simulink model "soc_dvbs2_fpga"  (R2025b)
settings: Solver=FixedStepDiscrete  StartTime=0.0  StopTime=0  RelTol=1e-3
InitFcn:
  | soc_dvbs2_init;
values from neighbouring files (symbols this model uses):
  Rsym = 4e6    (= 4000000)    [soc_dvbs2_init.m]
  soc_dvbs2_txPacketBits = [1 1 0 1 0 1 1 1 0 1 1 1 ... (2972 elements, 2972x1)]    [soc_dvbs2_txPacketBits.mat]
  syncWord = (dec2bin(hex2dec('AC')) - '0').'    [soc_dvbs2_init.m]
  txDataOut = txobj(frameBits(:))    [soc_dvbs2_init.m]
  txFiltCoeff = txobj.pTxFilterCoeff    [soc_dvbs2_init.m]
undefined symbols (not defined in the file or in its folder): Add, coefficientsLog, coefficientsSqrt1, coefficientsSqrt2, dataBits, designMultirateFIR, noisePow, NumBits1, NumBits2, seedsURNG1, seedsURNG2, Shift, Slope1, Slope2, soc_dvbs2_designFIRFilter, txDataOutS1, txDataOutS10, txDataOutS12, txDataOutS13, txDataOutS14, txDataOutS15, txDataOutS16, txDataOutS18, txDataOutS19, txDataOutS2, txDataOutS20, txDataOutS21, txDataOutS22, txDataOutS24, txDataOutS25, txDataOutS26, txDataOutS27, txDataOutS3, txDataOutS4, txDataOutS5, txDataOutS6, txDataOutS7, txDataOutS8, txDataOutS9
libraries: simulink x214, hdlsllib x211, dspsigops x22, dsphdlfiltering2 x8, dsphdlsigops2 x5, commseqgen3 x5, dsphdlmathfun2 x3, hwlogicconnlib x2, whdledac x2, commhdlcrc x2, whdlutilities x1, whdlmod x1
(part 11 of 12)

== system soc_dvbs2_fpga/DVBS2/DVBS2 TxRx/DVB-S2 HDL Receiver/Synchronizer and PL Header Decoder/Time Frequency and Coarse Phase Synchronizer/Fine Frequency Synchronizer/Modified L and R Algorithm/L and R Algorithm 18 point/Compute R(m) for 1 to 6/Compute R(m)_1/Complex Multiplier ==
  In1 : Inport
  In2 : Inport  Port=2
  AddADn : Sum  Inputs=++|  OutDataTypeStr=Inherit: Same as first input
  AddAUp : Sum  Inputs=|+-  OutDataTypeStr=Inherit: Same as first input
  AddBCtr : Sum  Inputs=+|+
  AddBDn : Sum  Inputs=|+-
  AddBUp : Sum  Inputs=++|
  Complex to Real-Imag : ComplexToRealImag
  Complex to Real-Imag1 : ComplexToRealImag
  Delay{1..5,8..20} (18 alike) : Delay  DelayLength=1
  Delay{6..7,21..27} (9 alike) : Delay
  Product : Product
  Product1 : Product
  Product2 : Product
  Real-Imag to Complex : RealImagToComplex
  Out1 : Outport  VectorParamsAs1DForOutWhenUnconnected=off
  wires:
  Delay27/1 -> Delay18/1
  Delay26/1 -> Delay17/1
  Delay25/1 -> Delay16/1
  Delay24/1 -> Product2/2
  Delay23/1 -> Product2/1
  Delay22/1 -> Product1/2
  Delay21/1 -> Product1/1
  Delay7/1 -> Product/2
  Delay6/1 -> Product/1
  In1/1 -> Complex to Real-Imag/1
  In2/1 -> Complex to Real-Imag1/1
  Complex to Real-Imag1/1 -> [RE2]
  Complex to Real-Imag1/2 -> [IM2]
  [IM2] -> Delay10/1
  [RE2] -> Delay9/1
  Complex to Real-Imag/1 -> Delay11/1
  AddBUp/1 -> Delay8/1
  [RE2] -> Delay14/1
  [IM2] -> Delay15/1
  AddBDn/1 -> Delay5/1
  Complex to Real-Imag/2 -> Delay13/1
  AddBCtr/1 -> Delay2/1
  [IM2] -> Delay12/1
  AddADn/1 -> Delay20/1
  AddAUp/1 -> Delay19/1
  Real-Imag to Complex/1 -> Out1/1
  Product/1 -> Delay25/1
  Product1/1 -> Delay26/1
  Product2/1 -> Delay27/1
  Delay5/1 -> Delay24/1
  Delay4/1 -> Delay23/1
  Delay3/1 -> Delay22/1
  Delay2/1 -> Delay21/1
  Delay8/1 -> Delay6/1
  Delay9/1 -> AddBUp/1
  Delay10/1 -> AddBUp/2
  Delay14/1 -> AddBDn/1
  Delay15/1 -> AddBDn/2
  Delay16/1 -> AddAUp/1
  Delay17/1 -> AddADn/1, AddAUp/2
  Delay18/1 -> AddADn/2
  Delay19/1 -> Real-Imag to Complex/1
  Delay20/1 -> Real-Imag to Complex/2
  Delay1/1 -> Delay7/1
  Delay11/1 -> AddBCtr/1, Delay1/1
  Delay12/1 -> Delay3/1
  Delay13/1 -> AddBCtr/2, Delay4/1

== system soc_dvbs2_fpga/DVBS2/DVBS2 TxRx/DVB-S2 HDL Receiver/Synchronizer and PL Header Decoder/Time Frequency and Coarse Phase Synchronizer/Fine Frequency Synchronizer/Modified L and R Algorithm/L and R Algorithm 18 point/Compute R(m) for 1 to 6/Compute R(m)_2/Complex Multiplier ==
  In1 : Inport
  In2 : Inport  Port=2
  AddADn : Sum  Inputs=++|  OutDataTypeStr=Inherit: Same as first input
  AddAUp : Sum  Inputs=|+-  OutDataTypeStr=Inherit: Same as first input
  AddBCtr : Sum  Inputs=+|+
  AddBDn : Sum  Inputs=|+-
  AddBUp : Sum  Inputs=++|
  Complex to Real-Imag : ComplexToRealImag
  Complex to Real-Imag1 : ComplexToRealImag
  Delay{1..5,8..20} (18 alike) : Delay  DelayLength=1
  Delay{6..7,21..27} (9 alike) : Delay
  Product : Product
  Product1 : Product
  Product2 : Product
  Real-Imag to Complex : RealImagToComplex
  Out1 : Outport  VectorParamsAs1DForOutWhenUnconnected=off
  wires:
  Delay13/1 -> Delay4/1, AddBCtr/2
  Delay12/1 -> Delay3/1
  Delay11/1 -> Delay1/1, AddBCtr/1
  Delay1/1 -> Delay7/1
  Delay20/1 -> Real-Imag to Complex/2
  Delay19/1 -> Real-Imag to Complex/1
  Delay18/1 -> AddADn/2
  Delay17/1 -> AddAUp/2, AddADn/1
  Delay16/1 -> AddAUp/1
  Delay15/1 -> AddBDn/2
  Delay14/1 -> AddBDn/1
  Delay10/1 -> AddBUp/2
  Delay9/1 -> AddBUp/1
  Delay8/1 -> Delay6/1
  Delay2/1 -> Delay21/1
  Delay3/1 -> Delay22/1
  Delay4/1 -> Delay23/1
  Delay5/1 -> Delay24/1
  Product2/1 -> Delay27/1
  Product1/1 -> Delay26/1
  Product/1 -> Delay25/1
  Real-Imag to Complex/1 -> Out1/1
  AddAUp/1 -> Delay19/1
  AddADn/1 -> Delay20/1
  [IM2] -> Delay12/1
  AddBCtr/1 -> Delay2/1
  Complex to Real-Imag/2 -> Delay13/1
  AddBDn/1 -> Delay5/1
  [IM2] -> Delay15/1
  [RE2] -> Delay14/1
  AddBUp/1 -> Delay8/1
  Complex to Real-Imag/1 -> Delay11/1
  [RE2] -> Delay9/1
  [IM2] -> Delay10/1
  Complex to Real-Imag1/2 -> [IM2]
  Complex to Real-Imag1/1 -> [RE2]
  In2/1 -> Complex to Real-Imag1/1
  In1/1 -> Complex to Real-Imag/1
  Delay6/1 -> Product/1
  Delay7/1 -> Product/2
  Delay21/1 -> Product1/1
  Delay22/1 -> Product1/2
  Delay23/1 -> Product2/1
  Delay24/1 -> Product2/2
  Delay25/1 -> Delay16/1
  Delay26/1 -> Delay17/1
  Delay27/1 -> Delay18/1

== system soc_dvbs2_fpga/DVBS2/DVBS2 TxRx/DVB-S2 HDL Receiver/Synchronizer and PL Header Decoder/Time Frequency and Coarse Phase Synchronizer/Fine Frequency Synchronizer/Modified L and R Algorithm/L and R Algorithm 18 point/Compute R(m) for 1 to 6/Compute R(m)_3/Complex Multiplier ==
  In1 : Inport
  In2 : Inport  Port=2
  AddADn : Sum  Inputs=++|  OutDataTypeStr=Inherit: Same as first input
  AddAUp : Sum  Inputs=|+-  OutDataTypeStr=Inherit: Same as first input
  AddBCtr : Sum  Inputs=+|+
  AddBDn : Sum  Inputs=|+-
  AddBUp : Sum  Inputs=++|
  Complex to Real-Imag : ComplexToRealImag
  Complex to Real-Imag1 : ComplexToRealImag
  Delay{1..5,8..20} (18 alike) : Delay  DelayLength=1
  Delay{6..7,21..27} (9 alike) : Delay
  Product : Product
  Product1 : Product
  Product2 : Product
  Real-Imag to Complex : RealImagToComplex
  Out1 : Outport  VectorParamsAs1DForOutWhenUnconnected=off
  wires:
  Delay27/1 -> Delay18/1
  Delay26/1 -> Delay17/1
  Delay25/1 -> Delay16/1
  Delay24/1 -> Product2/2
  Delay23/1 -> Product2/1
  Delay22/1 -> Product1/2
  Delay21/1 -> Product1/1
  Delay7/1 -> Product/2
  Delay6/1 -> Product/1
  In1/1 -> Complex to Real-Imag/1
  In2/1 -> Complex to Real-Imag1/1
  Complex to Real-Imag1/1 -> [RE2]
  Complex to Real-Imag1/2 -> [IM2]
  [IM2] -> Delay10/1
  [RE2] -> Delay9/1
  Complex to Real-Imag/1 -> Delay11/1
  AddBUp/1 -> Delay8/1
  [RE2] -> Delay14/1
  [IM2] -> Delay15/1
  AddBDn/1 -> Delay5/1
  Complex to Real-Imag/2 -> Delay13/1
  AddBCtr/1 -> Delay2/1
  [IM2] -> Delay12/1
  AddADn/1 -> Delay20/1
  AddAUp/1 -> Delay19/1
  Real-Imag to Complex/1 -> Out1/1
  Product/1 -> Delay25/1
  Product1/1 -> Delay26/1
  Product2/1 -> Delay27/1
  Delay5/1 -> Delay24/1
  Delay4/1 -> Delay23/1
  Delay3/1 -> Delay22/1
  Delay2/1 -> Delay21/1
  Delay8/1 -> Delay6/1
  Delay9/1 -> AddBUp/1
  Delay10/1 -> AddBUp/2
  Delay14/1 -> AddBDn/1
  Delay15/1 -> AddBDn/2
  Delay16/1 -> AddAUp/1
  Delay17/1 -> AddADn/1, AddAUp/2
  Delay18/1 -> AddADn/2
  Delay19/1 -> Real-Imag to Complex/1
  Delay20/1 -> Real-Imag to Complex/2
  Delay1/1 -> Delay7/1
  Delay11/1 -> AddBCtr/1, Delay1/1
  Delay12/1 -> Delay3/1
  Delay13/1 -> AddBCtr/2, Delay4/1

== system soc_dvbs2_fpga/DVBS2/DVBS2 TxRx/DVB-S2 HDL Receiver/Synchronizer and PL Header Decoder/Time Frequency and Coarse Phase Synchronizer/Fine Frequency Synchronizer/Modified L and R Algorithm/L and R Algorithm 18 point/Compute R(m) for 1 to 6/Compute R(m)_4/Complex Multiplier ==
  In1 : Inport
  In2 : Inport  Port=2
  AddADn : Sum  Inputs=++|  OutDataTypeStr=Inherit: Same as first input
  AddAUp : Sum  Inputs=|+-  OutDataTypeStr=Inherit: Same as first input
  AddBCtr : Sum  Inputs=+|+
  AddBDn : Sum  Inputs=|+-
  AddBUp : Sum  Inputs=++|
  Complex to Real-Imag : ComplexToRealImag
  Complex to Real-Imag1 : ComplexToRealImag
  Delay{1..5,8..20} (18 alike) : Delay  DelayLength=1
  Delay{6..7,21..27} (9 alike) : Delay
  Product : Product
  Product1 : Product
  Product2 : Product
  Real-Imag to Complex : RealImagToComplex
  Out1 : Outport  VectorParamsAs1DForOutWhenUnconnected=off
  wires:
  Delay13/1 -> Delay4/1, AddBCtr/2
  Delay12/1 -> Delay3/1
  Delay11/1 -> Delay1/1, AddBCtr/1
  Delay1/1 -> Delay7/1
  Delay20/1 -> Real-Imag to Complex/2
  Delay19/1 -> Real-Imag to Complex/1
  Delay18/1 -> AddADn/2
  Delay17/1 -> AddAUp/2, AddADn/1
  Delay16/1 -> AddAUp/1
  Delay15/1 -> AddBDn/2
  Delay14/1 -> AddBDn/1
  Delay10/1 -> AddBUp/2
  Delay9/1 -> AddBUp/1
  Delay8/1 -> Delay6/1
  Delay2/1 -> Delay21/1
  Delay3/1 -> Delay22/1
  Delay4/1 -> Delay23/1
  Delay5/1 -> Delay24/1
  Product2/1 -> Delay27/1
  Product1/1 -> Delay26/1
  Product/1 -> Delay25/1
  Real-Imag to Complex/1 -> Out1/1
  AddAUp/1 -> Delay19/1
  AddADn/1 -> Delay20/1
  [IM2] -> Delay12/1
  AddBCtr/1 -> Delay2/1
  Complex to Real-Imag/2 -> Delay13/1
  AddBDn/1 -> Delay5/1
  [IM2] -> Delay15/1
  [RE2] -> Delay14/1
  AddBUp/1 -> Delay8/1
  Complex to Real-Imag/1 -> Delay11/1
  [RE2] -> Delay9/1
  [IM2] -> Delay10/1
  Complex to Real-Imag1/2 -> [IM2]
  Complex to Real-Imag1/1 -> [RE2]
  In2/1 -> Complex to Real-Imag1/1
  In1/1 -> Complex to Real-Imag/1
  Delay6/1 -> Product/1
  Delay7/1 -> Product/2
  Delay21/1 -> Product1/1
  Delay22/1 -> Product1/2
  Delay23/1 -> Product2/1
  Delay24/1 -> Product2/2
  Delay25/1 -> Delay16/1
  Delay26/1 -> Delay17/1
  Delay27/1 -> Delay18/1

== system soc_dvbs2_fpga/DVBS2/DVBS2 TxRx/DVB-S2 HDL Receiver/Synchronizer and PL Header Decoder/Time Frequency and Coarse Phase Synchronizer/Fine Frequency Synchronizer/Modified L and R Algorithm/L and R Algorithm 18 point/Compute R(m) for 1 to 6/Compute R(m)_5/Complex Multiplier ==
  In1 : Inport
  In2 : Inport  Port=2
  AddADn : Sum  Inputs=++|  OutDataTypeStr=Inherit: Same as first input
  AddAUp : Sum  Inputs=|+-  OutDataTypeStr=Inherit: Same as first input
  AddBCtr : Sum  Inputs=+|+
  AddBDn : Sum  Inputs=|+-
  AddBUp : Sum  Inputs=++|
  Complex to Real-Imag : ComplexToRealImag
  Complex to Real-Imag1 : ComplexToRealImag
  Delay{1..5,8..20} (18 alike) : Delay  DelayLength=1
  Delay{6..7,21..27} (9 alike) : Delay
  Product : Product
  Product1 : Product
  Product2 : Product
  Real-Imag to Complex : RealImagToComplex
  Out1 : Outport  VectorParamsAs1DForOutWhenUnconnected=off
  wires:
  Delay27/1 -> Delay18/1
  Delay26/1 -> Delay17/1
  Delay25/1 -> Delay16/1
  Delay24/1 -> Product2/2
  Delay23/1 -> Product2/1
  Delay22/1 -> Product1/2
  Delay21/1 -> Product1/1
  Delay7/1 -> Product/2
  Delay6/1 -> Product/1
  In1/1 -> Complex to Real-Imag/1
  In2/1 -> Complex to Real-Imag1/1
  Complex to Real-Imag1/1 -> [RE2]
  Complex to Real-Imag1/2 -> [IM2]
  [IM2] -> Delay10/1
  [RE2] -> Delay9/1
  Complex to Real-Imag/1 -> Delay11/1
  AddBUp/1 -> Delay8/1
  [RE2] -> Delay14/1
  [IM2] -> Delay15/1
  AddBDn/1 -> Delay5/1
  Complex to Real-Imag/2 -> Delay13/1
  AddBCtr/1 -> Delay2/1
  [IM2] -> Delay12/1
  AddADn/1 -> Delay20/1
  AddAUp/1 -> Delay19/1
  Real-Imag to Complex/1 -> Out1/1
  Product/1 -> Delay25/1
  Product1/1 -> Delay26/1
  Product2/1 -> Delay27/1
  Delay5/1 -> Delay24/1
  Delay4/1 -> Delay23/1
  Delay3/1 -> Delay22/1
  Delay2/1 -> Delay21/1
  Delay8/1 -> Delay6/1
  Delay9/1 -> AddBUp/1
  Delay10/1 -> AddBUp/2
  Delay14/1 -> AddBDn/1
  Delay15/1 -> AddBDn/2
  Delay16/1 -> AddAUp/1
  Delay17/1 -> AddADn/1, AddAUp/2
  Delay18/1 -> AddADn/2
  Delay19/1 -> Real-Imag to Complex/1
  Delay20/1 -> Real-Imag to Complex/2
  Delay1/1 -> Delay7/1
  Delay11/1 -> AddBCtr/1, Delay1/1
  Delay12/1 -> Delay3/1
  Delay13/1 -> AddBCtr/2, Delay4/1

== system soc_dvbs2_fpga/DVBS2/DVBS2 TxRx/DVB-S2 HDL Receiver/Synchronizer and PL Header Decoder/Time Frequency and Coarse Phase Synchronizer/Fine Frequency Synchronizer/Modified L and R Algorithm/L and R Algorithm 18 point/Compute R(m) for 1 to 6/Compute R(m)_6/Complex Multiplier ==
  In1 : Inport
  In2 : Inport  Port=2
  AddADn : Sum  Inputs=++|  OutDataTypeStr=Inherit: Same as first input
  AddAUp : Sum  Inputs=|+-  OutDataTypeStr=Inherit: Same as first input
  AddBCtr : Sum  Inputs=+|+
  AddBDn : Sum  Inputs=|+-
  AddBUp : Sum  Inputs=++|
  Complex to Real-Imag : ComplexToRealImag
  Complex to Real-Imag1 : ComplexToRealImag
  Delay{1..5,8..20} (18 alike) : Delay  DelayLength=1
  Delay{6..7,21..27} (9 alike) : Delay
  Product : Product
  Product1 : Product
  Product2 : Product
  Real-Imag to Complex : RealImagToComplex
  Out1 : Outport  VectorParamsAs1DForOutWhenUnconnected=off
  wires:
  Delay13/1 -> Delay4/1, AddBCtr/2
  Delay12/1 -> Delay3/1
  Delay11/1 -> Delay1/1, AddBCtr/1
  Delay1/1 -> Delay7/1
  Delay20/1 -> Real-Imag to Complex/2
  Delay19/1 -> Real-Imag to Complex/1
  Delay18/1 -> AddADn/2
  Delay17/1 -> AddAUp/2, AddADn/1
  Delay16/1 -> AddAUp/1
  Delay15/1 -> AddBDn/2
  Delay14/1 -> AddBDn/1
  Delay10/1 -> AddBUp/2
  Delay9/1 -> AddBUp/1
  Delay8/1 -> Delay6/1
  Delay2/1 -> Delay21/1
  Delay3/1 -> Delay22/1
  Delay4/1 -> Delay23/1
  Delay5/1 -> Delay24/1
  Product2/1 -> Delay27/1
  Product1/1 -> Delay26/1
  Product/1 -> Delay25/1
  Real-Imag to Complex/1 -> Out1/1
  AddAUp/1 -> Delay19/1
  AddADn/1 -> Delay20/1
  [IM2] -> Delay12/1
  AddBCtr/1 -> Delay2/1
  Complex to Real-Imag/2 -> Delay13/1
  AddBDn/1 -> Delay5/1
  [IM2] -> Delay15/1
  [RE2] -> Delay14/1
  AddBUp/1 -> Delay8/1
  Complex to Real-Imag/1 -> Delay11/1
  [RE2] -> Delay9/1
  [IM2] -> Delay10/1
  Complex to Real-Imag1/2 -> [IM2]
  Complex to Real-Imag1/1 -> [RE2]
  In2/1 -> Complex to Real-Imag1/1
  In1/1 -> Complex to Real-Imag/1
  Delay6/1 -> Product/1
  Delay7/1 -> Product/2
  Delay21/1 -> Product1/1
  Delay22/1 -> Product1/2
  Delay23/1 -> Product2/1
  Delay24/1 -> Product2/2
  Delay25/1 -> Delay16/1
  Delay26/1 -> Delay17/1
  Delay27/1 -> Delay18/1

== system soc_dvbs2_fpga/DVBS2/DVBS2 TxRx/DVB-S2 HDL Receiver/Synchronizer and PL Header Decoder/Time Frequency and Coarse Phase Synchronizer/Fine Frequency Synchronizer/Modified L and R Algorithm/L and R Algorithm 18 point/Compute R(m) for 13 to 18/Compute R(m)_1/Complex Multiplier ==
  In1 : Inport
  In2 : Inport  Port=2
  AddADn : Sum  Inputs=++|  OutDataTypeStr=Inherit: Same as first input
  AddAUp : Sum  Inputs=|+-  OutDataTypeStr=Inherit: Same as first input
  AddBCtr : Sum  Inputs=+|+
  AddBDn : Sum  Inputs=|+-
  AddBUp : Sum  Inputs=++|
  Complex to Real-Imag : ComplexToRealImag
  Complex to Real-Imag1 : ComplexToRealImag
  Delay{1..5,8..20} (18 alike) : Delay  DelayLength=1
  Delay{6..7,21..27} (9 alike) : Delay
  Product : Product
  Product1 : Product
  Product2 : Product
  Real-Imag to Complex : RealImagToComplex
  Out1 : Outport  VectorParamsAs1DForOutWhenUnconnected=off
  wires:
  Delay27/1 -> Delay18/1
  Delay26/1 -> Delay17/1
  Delay25/1 -> Delay16/1
  Delay24/1 -> Product2/2
  Delay23/1 -> Product2/1
  Delay22/1 -> Product1/2
  Delay21/1 -> Product1/1
  Delay7/1 -> Product/2
  Delay6/1 -> Product/1
  In1/1 -> Complex to Real-Imag/1
  In2/1 -> Complex to Real-Imag1/1
  Complex to Real-Imag1/1 -> [RE2]
  Complex to Real-Imag1/2 -> [IM2]
  [IM2] -> Delay10/1
  [RE2] -> Delay9/1
  Complex to Real-Imag/1 -> Delay11/1
  AddBUp/1 -> Delay8/1
  [RE2] -> Delay14/1
  [IM2] -> Delay15/1
  AddBDn/1 -> Delay5/1
  Complex to Real-Imag/2 -> Delay13/1
  AddBCtr/1 -> Delay2/1
  [IM2] -> Delay12/1
  AddADn/1 -> Delay20/1
  AddAUp/1 -> Delay19/1
  Real-Imag to Complex/1 -> Out1/1
  Product/1 -> Delay25/1
  Product1/1 -> Delay26/1
  Product2/1 -> Delay27/1
  Delay5/1 -> Delay24/1
  Delay4/1 -> Delay23/1
  Delay3/1 -> Delay22/1
  Delay2/1 -> Delay21/1
  Delay8/1 -> Delay6/1
  Delay9/1 -> AddBUp/1
  Delay10/1 -> AddBUp/2
  Delay14/1 -> AddBDn/1
  Delay15/1 -> AddBDn/2
  Delay16/1 -> AddAUp/1
  Delay17/1 -> AddADn/1, AddAUp/2
  Delay18/1 -> AddADn/2
  Delay19/1 -> Real-Imag to Complex/1
  Delay20/1 -> Real-Imag to Complex/2
  Delay1/1 -> Delay7/1
  Delay11/1 -> AddBCtr/1, Delay1/1
  Delay12/1 -> Delay3/1
  Delay13/1 -> AddBCtr/2, Delay4/1

== system soc_dvbs2_fpga/DVBS2/DVBS2 TxRx/DVB-S2 HDL Receiver/Synchronizer and PL Header Decoder/Time Frequency and Coarse Phase Synchronizer/Fine Frequency Synchronizer/Modified L and R Algorithm/L and R Algorithm 18 point/Compute R(m) for 13 to 18/Compute R(m)_2/Complex Multiplier ==
  In1 : Inport
  In2 : Inport  Port=2
  AddADn : Sum  Inputs=++|  OutDataTypeStr=Inherit: Same as first input
  AddAUp : Sum  Inputs=|+-  OutDataTypeStr=Inherit: Same as first input
  AddBCtr : Sum  Inputs=+|+
  AddBDn : Sum  Inputs=|+-
  AddBUp : Sum  Inputs=++|
  Complex to Real-Imag : ComplexToRealImag
  Complex to Real-Imag1 : ComplexToRealImag
  Delay{1..5,8..20} (18 alike) : Delay  DelayLength=1
  Delay{6..7,21..27} (9 alike) : Delay
  Product : Product
  Product1 : Product
  Product2 : Product
  Real-Imag to Complex : RealImagToComplex
  Out1 : Outport  VectorParamsAs1DForOutWhenUnconnected=off
  wires:
  Delay13/1 -> Delay4/1, AddBCtr/2
  Delay12/1 -> Delay3/1
  Delay11/1 -> Delay1/1, AddBCtr/1
  Delay1/1 -> Delay7/1
  Delay20/1 -> Real-Imag to Complex/2
  Delay19/1 -> Real-Imag to Complex/1
  Delay18/1 -> AddADn/2
  Delay17/1 -> AddAUp/2, AddADn/1
  Delay16/1 -> AddAUp/1
  Delay15/1 -> AddBDn/2
  Delay14/1 -> AddBDn/1
  Delay10/1 -> AddBUp/2
  Delay9/1 -> AddBUp/1
  Delay8/1 -> Delay6/1
  Delay2/1 -> Delay21/1
  Delay3/1 -> Delay22/1
  Delay4/1 -> Delay23/1
  Delay5/1 -> Delay24/1
  Product2/1 -> Delay27/1
  Product1/1 -> Delay26/1
  Product/1 -> Delay25/1
  Real-Imag to Complex/1 -> Out1/1
  AddAUp/1 -> Delay19/1
  AddADn/1 -> Delay20/1
  [IM2] -> Delay12/1
  AddBCtr/1 -> Delay2/1
  Complex to Real-Imag/2 -> Delay13/1
  AddBDn/1 -> Delay5/1
  [IM2] -> Delay15/1
  [RE2] -> Delay14/1
  AddBUp/1 -> Delay8/1
  Complex to Real-Imag/1 -> Delay11/1
  [RE2] -> Delay9/1
  [IM2] -> Delay10/1
  Complex to Real-Imag1/2 -> [IM2]
  Complex to Real-Imag1/1 -> [RE2]
  In2/1 -> Complex to Real-Imag1/1
  In1/1 -> Complex to Real-Imag/1
  Delay6/1 -> Product/1
  Delay7/1 -> Product/2
  Delay21/1 -> Product1/1
  Delay22/1 -> Product1/2
  Delay23/1 -> Product2/1
  Delay24/1 -> Product2/2
  Delay25/1 -> Delay16/1
  Delay26/1 -> Delay17/1
  Delay27/1 -> Delay18/1

== system soc_dvbs2_fpga/DVBS2/DVBS2 TxRx/DVB-S2 HDL Receiver/Synchronizer and PL Header Decoder/Time Frequency and Coarse Phase Synchronizer/Fine Frequency Synchronizer/Modified L and R Algorithm/L and R Algorithm 18 point/Compute R(m) for 13 to 18/Compute R(m)_3/Complex Multiplier ==
  In1 : Inport
  In2 : Inport  Port=2
  AddADn : Sum  Inputs=++|  OutDataTypeStr=Inherit: Same as first input
  AddAUp : Sum  Inputs=|+-  OutDataTypeStr=Inherit: Same as first input
  AddBCtr : Sum  Inputs=+|+
  AddBDn : Sum  Inputs=|+-
  AddBUp : Sum  Inputs=++|
  Complex to Real-Imag : ComplexToRealImag
  Complex to Real-Imag1 : ComplexToRealImag
  Delay{1..5,8..20} (18 alike) : Delay  DelayLength=1
  Delay{6..7,21..27} (9 alike) : Delay
  Product : Product
  Product1 : Product
  Product2 : Product
  Real-Imag to Complex : RealImagToComplex
  Out1 : Outport  VectorParamsAs1DForOutWhenUnconnected=off
  wires:
  Delay27/1 -> Delay18/1
  Delay26/1 -> Delay17/1
  Delay25/1 -> Delay16/1
  Delay24/1 -> Product2/2
  Delay23/1 -> Product2/1
  Delay22/1 -> Product1/2
  Delay21/1 -> Product1/1
  Delay7/1 -> Product/2
  Delay6/1 -> Product/1
  In1/1 -> Complex to Real-Imag/1
  In2/1 -> Complex to Real-Imag1/1
  Complex to Real-Imag1/1 -> [RE2]
  Complex to Real-Imag1/2 -> [IM2]
  [IM2] -> Delay10/1
  [RE2] -> Delay9/1
  Complex to Real-Imag/1 -> Delay11/1
  AddBUp/1 -> Delay8/1
  [RE2] -> Delay14/1
  [IM2] -> Delay15/1
  AddBDn/1 -> Delay5/1
  Complex to Real-Imag/2 -> Delay13/1
  AddBCtr/1 -> Delay2/1
  [IM2] -> Delay12/1
  AddADn/1 -> Delay20/1
  AddAUp/1 -> Delay19/1
  Real-Imag to Complex/1 -> Out1/1
  Product/1 -> Delay25/1
  Product1/1 -> Delay26/1
  Product2/1 -> Delay27/1
  Delay5/1 -> Delay24/1
  Delay4/1 -> Delay23/1
  Delay3/1 -> Delay22/1
  Delay2/1 -> Delay21/1
  Delay8/1 -> Delay6/1
  Delay9/1 -> AddBUp/1
  Delay10/1 -> AddBUp/2
  Delay14/1 -> AddBDn/1
  Delay15/1 -> AddBDn/2
  Delay16/1 -> AddAUp/1
  Delay17/1 -> AddADn/1, AddAUp/2
  Delay18/1 -> AddADn/2
  Delay19/1 -> Real-Imag to Complex/1
  Delay20/1 -> Real-Imag to Complex/2
  Delay1/1 -> Delay7/1
  Delay11/1 -> AddBCtr/1, Delay1/1
  Delay12/1 -> Delay3/1
  Delay13/1 -> AddBCtr/2, Delay4/1

== system soc_dvbs2_fpga/DVBS2/DVBS2 TxRx/DVB-S2 HDL Receiver/Synchronizer and PL Header Decoder/Time Frequency and Coarse Phase Synchronizer/Fine Frequency Synchronizer/Modified L and R Algorithm/L and R Algorithm 18 point/Compute R(m) for 13 to 18/Compute R(m)_4/Complex Multiplier ==
  In1 : Inport
  In2 : Inport  Port=2
  AddADn : Sum  Inputs=++|  OutDataTypeStr=Inherit: Same as first input
  AddAUp : Sum  Inputs=|+-  OutDataTypeStr=Inherit: Same as first input
  AddBCtr : Sum  Inputs=+|+
  AddBDn : Sum  Inputs=|+-
  AddBUp : Sum  Inputs=++|
  Complex to Real-Imag : ComplexToRealImag
  Complex to Real-Imag1 : ComplexToRealImag
  Delay{1..5,8..20} (18 alike) : Delay  DelayLength=1
  Delay{6..7,21..27} (9 alike) : Delay
  Product : Product
  Product1 : Product
  Product2 : Product
  Real-Imag to Complex : RealImagToComplex
  Out1 : Outport  VectorParamsAs1DForOutWhenUnconnected=off
  wires:
  Delay13/1 -> Delay4/1, AddBCtr/2
  Delay12/1 -> Delay3/1
  Delay11/1 -> Delay1/1, AddBCtr/1
  Delay1/1 -> Delay7/1
  Delay20/1 -> Real-Imag to Complex/2
  Delay19/1 -> Real-Imag to Complex/1
  Delay18/1 -> AddADn/2
  Delay17/1 -> AddAUp/2, AddADn/1
  Delay16/1 -> AddAUp/1
  Delay15/1 -> AddBDn/2
  Delay14/1 -> AddBDn/1
  Delay10/1 -> AddBUp/2
  Delay9/1 -> AddBUp/1
  Delay8/1 -> Delay6/1
  Delay2/1 -> Delay21/1
  Delay3/1 -> Delay22/1
  Delay4/1 -> Delay23/1
  Delay5/1 -> Delay24/1
  Product2/1 -> Delay27/1
  Product1/1 -> Delay26/1
  Product/1 -> Delay25/1
  Real-Imag to Complex/1 -> Out1/1
  AddAUp/1 -> Delay19/1
  AddADn/1 -> Delay20/1
  [IM2] -> Delay12/1
  AddBCtr/1 -> Delay2/1
  Complex to Real-Imag/2 -> Delay13/1
  AddBDn/1 -> Delay5/1
  [IM2] -> Delay15/1
  [RE2] -> Delay14/1
  AddBUp/1 -> Delay8/1
  Complex to Real-Imag/1 -> Delay11/1
  [RE2] -> Delay9/1
  [IM2] -> Delay10/1
  Complex to Real-Imag1/2 -> [IM2]
  Complex to Real-Imag1/1 -> [RE2]
  In2/1 -> Complex to Real-Imag1/1
  In1/1 -> Complex to Real-Imag/1
  Delay6/1 -> Product/1
  Delay7/1 -> Product/2
  Delay21/1 -> Product1/1
  Delay22/1 -> Product1/2
  Delay23/1 -> Product2/1
  Delay24/1 -> Product2/2
  Delay25/1 -> Delay16/1
  Delay26/1 -> Delay17/1
  Delay27/1 -> Delay18/1

== system soc_dvbs2_fpga/DVBS2/DVBS2 TxRx/DVB-S2 HDL Receiver/Synchronizer and PL Header Decoder/Time Frequency and Coarse Phase Synchronizer/Fine Frequency Synchronizer/Modified L and R Algorithm/L and R Algorithm 18 point/Compute R(m) for 13 to 18/Compute R(m)_5/Complex Multiplier ==
  In1 : Inport
  In2 : Inport  Port=2
  AddADn : Sum  Inputs=++|  OutDataTypeStr=Inherit: Same as first input
  AddAUp : Sum  Inputs=|+-  OutDataTypeStr=Inherit: Same as first input
  AddBCtr : Sum  Inputs=+|+
  AddBDn : Sum  Inputs=|+-
  AddBUp : Sum  Inputs=++|
  Complex to Real-Imag : ComplexToRealImag
  Complex to Real-Imag1 : ComplexToRealImag
  Delay{1..5,8..20} (18 alike) : Delay  DelayLength=1
  Delay{6..7,21..27} (9 alike) : Delay
  Product : Product
  Product1 : Product
  Product2 : Product
  Real-Imag to Complex : RealImagToComplex
  Out1 : Outport  VectorParamsAs1DForOutWhenUnconnected=off
  wires:
  Delay27/1 -> Delay18/1
  Delay26/1 -> Delay17/1
  Delay25/1 -> Delay16/1
  Delay24/1 -> Product2/2
  Delay23/1 -> Product2/1
  Delay22/1 -> Product1/2
  Delay21/1 -> Product1/1
  Delay7/1 -> Product/2
  Delay6/1 -> Product/1
  In1/1 -> Complex to Real-Imag/1
  In2/1 -> Complex to Real-Imag1/1
  Complex to Real-Imag1/1 -> [RE2]
  Complex to Real-Imag1/2 -> [IM2]
  [IM2] -> Delay10/1
  [RE2] -> Delay9/1
  Complex to Real-Imag/1 -> Delay11/1
  AddBUp/1 -> Delay8/1
  [RE2] -> Delay14/1
  [IM2] -> Delay15/1
  AddBDn/1 -> Delay5/1
  Complex to Real-Imag/2 -> Delay13/1
  AddBCtr/1 -> Delay2/1
  [IM2] -> Delay12/1
  AddADn/1 -> Delay20/1
  AddAUp/1 -> Delay19/1
  Real-Imag to Complex/1 -> Out1/1
  Product/1 -> Delay25/1
  Product1/1 -> Delay26/1
  Product2/1 -> Delay27/1
  Delay5/1 -> Delay24/1
  Delay4/1 -> Delay23/1
  Delay3/1 -> Delay22/1
  Delay2/1 -> Delay21/1
  Delay8/1 -> Delay6/1
  Delay9/1 -> AddBUp/1
  Delay10/1 -> AddBUp/2
  Delay14/1 -> AddBDn/1
  Delay15/1 -> AddBDn/2
  Delay16/1 -> AddAUp/1
  Delay17/1 -> AddADn/1, AddAUp/2
  Delay18/1 -> AddADn/2
  Delay19/1 -> Real-Imag to Complex/1
  Delay20/1 -> Real-Imag to Complex/2
  Delay1/1 -> Delay7/1
  Delay11/1 -> AddBCtr/1, Delay1/1
  Delay12/1 -> Delay3/1
  Delay13/1 -> AddBCtr/2, Delay4/1

== system soc_dvbs2_fpga/DVBS2/DVBS2 TxRx/DVB-S2 HDL Receiver/Synchronizer and PL Header Decoder/Time Frequency and Coarse Phase Synchronizer/Fine Frequency Synchronizer/Modified L and R Algorithm/L and R Algorithm 18 point/Compute R(m) for 13 to 18/Compute R(m)_6/Complex Multiplier ==
  In1 : Inport
  In2 : Inport  Port=2
  AddADn : Sum  Inputs=++|  OutDataTypeStr=Inherit: Same as first input
  AddAUp : Sum  Inputs=|+-  OutDataTypeStr=Inherit: Same as first input
  AddBCtr : Sum  Inputs=+|+
  AddBDn : Sum  Inputs=|+-
  AddBUp : Sum  Inputs=++|
  Complex to Real-Imag : ComplexToRealImag
  Complex to Real-Imag1 : ComplexToRealImag
  Delay{1..5,8..20} (18 alike) : Delay  DelayLength=1
  Delay{6..7,21..27} (9 alike) : Delay
  Product : Product
  Product1 : Product
  Product2 : Product
  Real-Imag to Complex : RealImagToComplex
  Out1 : Outport  VectorParamsAs1DForOutWhenUnconnected=off
  wires:
  Delay13/1 -> Delay4/1, AddBCtr/2
  Delay12/1 -> Delay3/1
  Delay11/1 -> Delay1/1, AddBCtr/1
  Delay1/1 -> Delay7/1
  Delay20/1 -> Real-Imag to Complex/2
  Delay19/1 -> Real-Imag to Complex/1
  Delay18/1 -> AddADn/2
  Delay17/1 -> AddAUp/2, AddADn/1
  Delay16/1 -> AddAUp/1
  Delay15/1 -> AddBDn/2
  Delay14/1 -> AddBDn/1
  Delay10/1 -> AddBUp/2
  Delay9/1 -> AddBUp/1
  Delay8/1 -> Delay6/1
  Delay2/1 -> Delay21/1
  Delay3/1 -> Delay22/1
  Delay4/1 -> Delay23/1
  Delay5/1 -> Delay24/1
  Product2/1 -> Delay27/1
  Product1/1 -> Delay26/1
  Product/1 -> Delay25/1
  Real-Imag to Complex/1 -> Out1/1
  AddAUp/1 -> Delay19/1
  AddADn/1 -> Delay20/1
  [IM2] -> Delay12/1
  AddBCtr/1 -> Delay2/1
  Complex to Real-Imag/2 -> Delay13/1
  AddBDn/1 -> Delay5/1
  [IM2] -> Delay15/1
  [RE2] -> Delay14/1
  AddBUp/1 -> Delay8/1
  Complex to Real-Imag/1 -> Delay11/1
  [RE2] -> Delay9/1
  [IM2] -> Delay10/1
  Complex to Real-Imag1/2 -> [IM2]
  Complex to Real-Imag1/1 -> [RE2]
  In2/1 -> Complex to Real-Imag1/1
  In1/1 -> Complex to Real-Imag/1
  Delay6/1 -> Product/1
  Delay7/1 -> Product/2
  Delay21/1 -> Product1/1
  Delay22/1 -> Product1/2
  Delay23/1 -> Product2/1
  Delay24/1 -> Product2/2
  Delay25/1 -> Delay16/1
  Delay26/1 -> Delay17/1
  Delay27/1 -> Delay18/1

== system soc_dvbs2_fpga/DVBS2/DVBS2 TxRx/DVB-S2 HDL Receiver/Synchronizer and PL Header Decoder/Time Frequency and Coarse Phase Synchronizer/Fine Frequency Synchronizer/Modified L and R Algorithm/L and R Algorithm 18 point/Compute R(m) for 7 to 12/Compute R(m)_1/Complex Multiplier ==
  In1 : Inport
  In2 : Inport  Port=2
  AddADn : Sum  Inputs=++|  OutDataTypeStr=Inherit: Same as first input
  AddAUp : Sum  Inputs=|+-  OutDataTypeStr=Inherit: Same as first input
  AddBCtr : Sum  Inputs=+|+
  AddBDn : Sum  Inputs=|+-
  AddBUp : Sum  Inputs=++|
  Complex to Real-Imag : ComplexToRealImag
  Complex to Real-Imag1 : ComplexToRealImag
  Delay{1..5,8..20} (18 alike) : Delay  DelayLength=1
  Delay{6..7,21..27} (9 alike) : Delay
  Product : Product
  Product1 : Product
  Product2 : Product
  Real-Imag to Complex : RealImagToComplex
  Out1 : Outport  VectorParamsAs1DForOutWhenUnconnected=off
  wires:
  Delay13/1 -> Delay4/1, AddBCtr/2
  Delay12/1 -> Delay3/1
  Delay11/1 -> Delay1/1, AddBCtr/1
  Delay1/1 -> Delay7/1
  Delay20/1 -> Real-Imag to Complex/2
  Delay19/1 -> Real-Imag to Complex/1
  Delay18/1 -> AddADn/2
  Delay17/1 -> AddAUp/2, AddADn/1
  Delay16/1 -> AddAUp/1
  Delay15/1 -> AddBDn/2
  Delay14/1 -> AddBDn/1
  Delay10/1 -> AddBUp/2
  Delay9/1 -> AddBUp/1
  Delay8/1 -> Delay6/1
  Delay2/1 -> Delay21/1
  Delay3/1 -> Delay22/1
  Delay4/1 -> Delay23/1
  Delay5/1 -> Delay24/1
  Product2/1 -> Delay27/1
  Product1/1 -> Delay26/1
  Product/1 -> Delay25/1
  Real-Imag to Complex/1 -> Out1/1
  AddAUp/1 -> Delay19/1
  AddADn/1 -> Delay20/1
  [IM2] -> Delay12/1
  AddBCtr/1 -> Delay2/1
  Complex to Real-Imag/2 -> Delay13/1
  AddBDn/1 -> Delay5/1
  [IM2] -> Delay15/1
  [RE2] -> Delay14/1
  AddBUp/1 -> Delay8/1
  Complex to Real-Imag/1 -> Delay11/1
  [RE2] -> Delay9/1
  [IM2] -> Delay10/1
  Complex to Real-Imag1/2 -> [IM2]
  Complex to Real-Imag1/1 -> [RE2]
  In2/1 -> Complex to Real-Imag1/1
  In1/1 -> Complex to Real-Imag/1
  Delay6/1 -> Product/1
  Delay7/1 -> Product/2
  Delay21/1 -> Product1/1
  Delay22/1 -> Product1/2
  Delay23/1 -> Product2/1
  Delay24/1 -> Product2/2
  Delay25/1 -> Delay16/1
  Delay26/1 -> Delay17/1
  Delay27/1 -> Delay18/1

== system soc_dvbs2_fpga/DVBS2/DVBS2 TxRx/DVB-S2 HDL Receiver/Synchronizer and PL Header Decoder/Time Frequency and Coarse Phase Synchronizer/Fine Frequency Synchronizer/Modified L and R Algorithm/L and R Algorithm 18 point/Compute R(m) for 7 to 12/Compute R(m)_2/Complex Multiplier ==
  In1 : Inport
  In2 : Inport  Port=2
  AddADn : Sum  Inputs=++|  OutDataTypeStr=Inherit: Same as first input
  AddAUp : Sum  Inputs=|+-  OutDataTypeStr=Inherit: Same as first input
  AddBCtr : Sum  Inputs=+|+
  AddBDn : Sum  Inputs=|+-
  AddBUp : Sum  Inputs=++|
  Complex to Real-Imag : ComplexToRealImag
  Complex to Real-Imag1 : ComplexToRealImag
  Delay{1..5,8..20} (18 alike) : Delay  DelayLength=1
  Delay{6..7,21..27} (9 alike) : Delay
  Product : Product
  Product1 : Product
  Product2 : Product
  Real-Imag to Complex : RealImagToComplex
  Out1 : Outport  VectorParamsAs1DForOutWhenUnconnected=off
  wires:
  Delay27/1 -> Delay18/1
  Delay26/1 -> Delay17/1
  Delay25/1 -> Delay16/1
  Delay24/1 -> Product2/2
  Delay23/1 -> Product2/1
  Delay22/1 -> Product1/2
  Delay21/1 -> Product1/1
  Delay7/1 -> Product/2
  Delay6/1 -> Product/1
  In1/1 -> Complex to Real-Imag/1
  In2/1 -> Complex to Real-Imag1/1
  Complex to Real-Imag1/1 -> [RE2]
  Complex to Real-Imag1/2 -> [IM2]
  [IM2] -> Delay10/1
  [RE2] -> Delay9/1
  Complex to Real-Imag/1 -> Delay11/1
  AddBUp/1 -> Delay8/1
  [RE2] -> Delay14/1
  [IM2] -> Delay15/1
  AddBDn/1 -> Delay5/1
  Complex to Real-Imag/2 -> Delay13/1
  AddBCtr/1 -> Delay2/1
  [IM2] -> Delay12/1
  AddADn/1 -> Delay20/1
  AddAUp/1 -> Delay19/1
  Real-Imag to Complex/1 -> Out1/1
  Product/1 -> Delay25/1
  Product1/1 -> Delay26/1
  Product2/1 -> Delay27/1
  Delay5/1 -> Delay24/1
  Delay4/1 -> Delay23/1
  Delay3/1 -> Delay22/1
  Delay2/1 -> Delay21/1
  Delay8/1 -> Delay6/1
  Delay9/1 -> AddBUp/1
  Delay10/1 -> AddBUp/2
  Delay14/1 -> AddBDn/1
  Delay15/1 -> AddBDn/2
  Delay16/1 -> AddAUp/1
  Delay17/1 -> AddADn/1, AddAUp/2
  Delay18/1 -> AddADn/2
  Delay19/1 -> Real-Imag to Complex/1
  Delay20/1 -> Real-Imag to Complex/2
  Delay1/1 -> Delay7/1
  Delay11/1 -> AddBCtr/1, Delay1/1
  Delay12/1 -> Delay3/1
  Delay13/1 -> AddBCtr/2, Delay4/1

== system soc_dvbs2_fpga/DVBS2/DVBS2 TxRx/DVB-S2 HDL Receiver/Synchronizer and PL Header Decoder/Time Frequency and Coarse Phase Synchronizer/Fine Frequency Synchronizer/Modified L and R Algorithm/L and R Algorithm 18 point/Compute R(m) for 7 to 12/Compute R(m)_3/Complex Multiplier ==
  In1 : Inport
  In2 : Inport  Port=2
  AddADn : Sum  Inputs=++|  OutDataTypeStr=Inherit: Same as first input
  AddAUp : Sum  Inputs=|+-  OutDataTypeStr=Inherit: Same as first input
  AddBCtr : Sum  Inputs=+|+
  AddBDn : Sum  Inputs=|+-
  AddBUp : Sum  Inputs=++|
  Complex to Real-Imag : ComplexToRealImag
  Complex to Real-Imag1 : ComplexToRealImag
  Delay{1..5,8..20} (18 alike) : Delay  DelayLength=1
  Delay{6..7,21..27} (9 alike) : Delay
  Product : Product
  Product1 : Product
  Product2 : Product
  Real-Imag to Complex : RealImagToComplex
  Out1 : Outport  VectorParamsAs1DForOutWhenUnconnected=off
  wires:
  Delay13/1 -> Delay4/1, AddBCtr/2
  Delay12/1 -> Delay3/1
  Delay11/1 -> Delay1/1, AddBCtr/1
  Delay1/1 -> Delay7/1
  Delay20/1 -> Real-Imag to Complex/2
  Delay19/1 -> Real-Imag to Complex/1
  Delay18/1 -> AddADn/2
  Delay17/1 -> AddAUp/2, AddADn/1
  Delay16/1 -> AddAUp/1
  Delay15/1 -> AddBDn/2
  Delay14/1 -> AddBDn/1
  Delay10/1 -> AddBUp/2
  Delay9/1 -> AddBUp/1
  Delay8/1 -> Delay6/1
  Delay2/1 -> Delay21/1
  Delay3/1 -> Delay22/1
  Delay4/1 -> Delay23/1
  Delay5/1 -> Delay24/1
  Product2/1 -> Delay27/1
  Product1/1 -> Delay26/1
  Product/1 -> Delay25/1
  Real-Imag to Complex/1 -> Out1/1
  AddAUp/1 -> Delay19/1
  AddADn/1 -> Delay20/1
  [IM2] -> Delay12/1
  AddBCtr/1 -> Delay2/1
  Complex to Real-Imag/2 -> Delay13/1
  AddBDn/1 -> Delay5/1
  [IM2] -> Delay15/1
  [RE2] -> Delay14/1
  AddBUp/1 -> Delay8/1
  Complex to Real-Imag/1 -> Delay11/1
  [RE2] -> Delay9/1
  [IM2] -> Delay10/1
  Complex to Real-Imag1/2 -> [IM2]
  Complex to Real-Imag1/1 -> [RE2]
  In2/1 -> Complex to Real-Imag1/1
  In1/1 -> Complex to Real-Imag/1
  Delay6/1 -> Product/1
  Delay7/1 -> Product/2
  Delay21/1 -> Product1/1
  Delay22/1 -> Product1/2
  Delay23/1 -> Product2/1
  Delay24/1 -> Product2/2
  Delay25/1 -> Delay16/1
  Delay26/1 -> Delay17/1
  Delay27/1 -> Delay18/1

== system soc_dvbs2_fpga/DVBS2/DVBS2 TxRx/DVB-S2 HDL Receiver/Synchronizer and PL Header Decoder/Time Frequency and Coarse Phase Synchronizer/Fine Frequency Synchronizer/Modified L and R Algorithm/L and R Algorithm 18 point/Compute R(m) for 7 to 12/Compute R(m)_4/Complex Multiplier ==
  In1 : Inport
  In2 : Inport  Port=2
  AddADn : Sum  Inputs=++|  OutDataTypeStr=Inherit: Same as first input
  AddAUp : Sum  Inputs=|+-  OutDataTypeStr=Inherit: Same as first input
  AddBCtr : Sum  Inputs=+|+
  AddBDn : Sum  Inputs=|+-
  AddBUp : Sum  Inputs=++|
  Complex to Real-Imag : ComplexToRealImag
  Complex to Real-Imag1 : ComplexToRealImag
  Delay{1..5,8..20} (18 alike) : Delay  DelayLength=1
  Delay{6..7,21..27} (9 alike) : Delay
  Product : Product
  Product1 : Product
  Product2 : Product
  Real-Imag to Complex : RealImagToComplex
  Out1 : Outport  VectorParamsAs1DForOutWhenUnconnected=off
  wires:
  Delay27/1 -> Delay18/1
  Delay26/1 -> Delay17/1
  Delay25/1 -> Delay16/1
  Delay24/1 -> Product2/2
  Delay23/1 -> Product2/1
  Delay22/1 -> Product1/2
  Delay21/1 -> Product1/1
  Delay7/1 -> Product/2
  Delay6/1 -> Product/1
  In1/1 -> Complex to Real-Imag/1
  In2/1 -> Complex to Real-Imag1/1
  Complex to Real-Imag1/1 -> [RE2]
  Complex to Real-Imag1/2 -> [IM2]
  [IM2] -> Delay10/1
  [RE2] -> Delay9/1
  Complex to Real-Imag/1 -> Delay11/1
  AddBUp/1 -> Delay8/1
  [RE2] -> Delay14/1
  [IM2] -> Delay15/1
  AddBDn/1 -> Delay5/1
  Complex to Real-Imag/2 -> Delay13/1
  AddBCtr/1 -> Delay2/1
  [IM2] -> Delay12/1
  AddADn/1 -> Delay20/1
  AddAUp/1 -> Delay19/1
  Real-Imag to Complex/1 -> Out1/1
  Product/1 -> Delay25/1
  Product1/1 -> Delay26/1
  Product2/1 -> Delay27/1
  Delay5/1 -> Delay24/1
  Delay4/1 -> Delay23/1
  Delay3/1 -> Delay22/1
  Delay2/1 -> Delay21/1
  Delay8/1 -> Delay6/1
  Delay9/1 -> AddBUp/1
  Delay10/1 -> AddBUp/2
  Delay14/1 -> AddBDn/1
  Delay15/1 -> AddBDn/2
  Delay16/1 -> AddAUp/1
  Delay17/1 -> AddADn/1, AddAUp/2
  Delay18/1 -> AddADn/2
  Delay19/1 -> Real-Imag to Complex/1
  Delay20/1 -> Real-Imag to Complex/2
  Delay1/1 -> Delay7/1
  Delay11/1 -> AddBCtr/1, Delay1/1
  Delay12/1 -> Delay3/1
  Delay13/1 -> AddBCtr/2, Delay4/1

== system soc_dvbs2_fpga/DVBS2/DVBS2 TxRx/DVB-S2 HDL Receiver/Synchronizer and PL Header Decoder/Time Frequency and Coarse Phase Synchronizer/Fine Frequency Synchronizer/Modified L and R Algorithm/L and R Algorithm 18 point/Compute R(m) for 7 to 12/Compute R(m)_5/Complex Multiplier ==
  In1 : Inport
  In2 : Inport  Port=2
  AddADn : Sum  Inputs=++|  OutDataTypeStr=Inherit: Same as first input
  AddAUp : Sum  Inputs=|+-  OutDataTypeStr=Inherit: Same as first input
  AddBCtr : Sum  Inputs=+|+
  AddBDn : Sum  Inputs=|+-
  AddBUp : Sum  Inputs=++|
  Complex to Real-Imag : ComplexToRealImag
  Complex to Real-Imag1 : ComplexToRealImag
  Delay{1..5,8..20} (18 alike) : Delay  DelayLength=1
  Delay{6..7,21..27} (9 alike) : Delay
  Product : Product
  Product1 : Product
  Product2 : Product
  Real-Imag to Complex : RealImagToComplex
  Out1 : Outport  VectorParamsAs1DForOutWhenUnconnected=off
  wires:
  Delay13/1 -> Delay4/1, AddBCtr/2
  Delay12/1 -> Delay3/1
  Delay11/1 -> Delay1/1, AddBCtr/1
  Delay1/1 -> Delay7/1
  Delay20/1 -> Real-Imag to Complex/2
  Delay19/1 -> Real-Imag to Complex/1
  Delay18/1 -> AddADn/2
  Delay17/1 -> AddAUp/2, AddADn/1
  Delay16/1 -> AddAUp/1
  Delay15/1 -> AddBDn/2
  Delay14/1 -> AddBDn/1
  Delay10/1 -> AddBUp/2
  Delay9/1 -> AddBUp/1
  Delay8/1 -> Delay6/1
  Delay2/1 -> Delay21/1
  Delay3/1 -> Delay22/1
  Delay4/1 -> Delay23/1
  Delay5/1 -> Delay24/1
  Product2/1 -> Delay27/1
  Product1/1 -> Delay26/1
  Product/1 -> Delay25/1
  Real-Imag to Complex/1 -> Out1/1
  AddAUp/1 -> Delay19/1
  AddADn/1 -> Delay20/1
  [IM2] -> Delay12/1
  AddBCtr/1 -> Delay2/1
  Complex to Real-Imag/2 -> Delay13/1
  AddBDn/1 -> Delay5/1
  [IM2] -> Delay15/1
  [RE2] -> Delay14/1
  AddBUp/1 -> Delay8/1
  Complex to Real-Imag/1 -> Delay11/1
  [RE2] -> Delay9/1
  [IM2] -> Delay10/1
  Complex to Real-Imag1/2 -> [IM2]
  Complex to Real-Imag1/1 -> [RE2]
  In2/1 -> Complex to Real-Imag1/1
  In1/1 -> Complex to Real-Imag/1
  Delay6/1 -> Product/1
  Delay7/1 -> Product/2
  Delay21/1 -> Product1/1
  Delay22/1 -> Product1/2
  Delay23/1 -> Product2/1
  Delay24/1 -> Product2/2
  Delay25/1 -> Delay16/1
  Delay26/1 -> Delay17/1
  Delay27/1 -> Delay18/1

== system soc_dvbs2_fpga/DVBS2/DVBS2 TxRx/DVB-S2 HDL Receiver/Synchronizer and PL Header Decoder/Time Frequency and Coarse Phase Synchronizer/Fine Frequency Synchronizer/Modified L and R Algorithm/L and R Algorithm 18 point/Compute R(m) for 7 to 12/Compute R(m)_6/Complex Multiplier ==
  In1 : Inport
  In2 : Inport  Port=2
  AddADn : Sum  Inputs=++|  OutDataTypeStr=Inherit: Same as first input
  AddAUp : Sum  Inputs=|+-  OutDataTypeStr=Inherit: Same as first input
  AddBCtr : Sum  Inputs=+|+
  AddBDn : Sum  Inputs=|+-
  AddBUp : Sum  Inputs=++|
  Complex to Real-Imag : ComplexToRealImag
  Complex to Real-Imag1 : ComplexToRealImag
  Delay{1..5,8..20} (18 alike) : Delay  DelayLength=1
  Delay{6..7,21..27} (9 alike) : Delay
  Product : Product
  Product1 : Product
  Product2 : Product
  Real-Imag to Complex : RealImagToComplex
  Out1 : Outport  VectorParamsAs1DForOutWhenUnconnected=off
  wires:
  Delay27/1 -> Delay18/1
  Delay26/1 -> Delay17/1
  Delay25/1 -> Delay16/1
  Delay24/1 -> Product2/2
  Delay23/1 -> Product2/1
  Delay22/1 -> Product1/2
  Delay21/1 -> Product1/1
  Delay7/1 -> Product/2
  Delay6/1 -> Product/1
  In1/1 -> Complex to Real-Imag/1
  In2/1 -> Complex to Real-Imag1/1
  Complex to Real-Imag1/1 -> [RE2]
  Complex to Real-Imag1/2 -> [IM2]
  [IM2] -> Delay10/1
  [RE2] -> Delay9/1
  Complex to Real-Imag/1 -> Delay11/1
  AddBUp/1 -> Delay8/1
  [RE2] -> Delay14/1
  [IM2] -> Delay15/1
  AddBDn/1 -> Delay5/1
  Complex to Real-Imag/2 -> Delay13/1
  AddBCtr/1 -> Delay2/1
  [IM2] -> Delay12/1
  AddADn/1 -> Delay20/1
  AddAUp/1 -> Delay19/1
  Real-Imag to Complex/1 -> Out1/1
  Product/1 -> Delay25/1
  Product1/1 -> Delay26/1
  Product2/1 -> Delay27/1
  Delay5/1 -> Delay24/1
  Delay4/1 -> Delay23/1
  Delay3/1 -> Delay22/1
  Delay2/1 -> Delay21/1
  Delay8/1 -> Delay6/1
  Delay9/1 -> AddBUp/1
  Delay10/1 -> AddBUp/2
  Delay14/1 -> AddBDn/1
  Delay15/1 -> AddBDn/2
  Delay16/1 -> AddAUp/1
  Delay17/1 -> AddADn/1, AddAUp/2
  Delay18/1 -> AddADn/2
  Delay19/1 -> Real-Imag to Complex/1
  Delay20/1 -> Real-Imag to Complex/2
  Delay1/1 -> Delay7/1
  Delay11/1 -> AddBCtr/1, Delay1/1
  Delay12/1 -> Delay3/1
  Delay13/1 -> AddBCtr/2, Delay4/1

== matlab function soc_dvbs2_fpga/DVBS2/DVBS2 TxRx/DVB-S2 HDL Receiver/Synchronizer and PL Header Decoder/Time Frequency and Coarse Phase Synchronizer/Time and Coarse Frequency Synchronizer/Symbol Synchronizer/Rate Handle/monostable ==
  data: trigger input; out output; nClocks parameter
function out = MonoStable(trigger,nClocks)
%#codegen

 persistent count;

 if isempty(count)
     count = fi(0,0,floor(log2(nClocks))+1,0,hdlfimath);
 end
 
 out = (count > 0);
 
 if (count > 0)
     count(:) = count - 1;
 end

 if trigger
     count(:) =  nClocks;
 end
 
end

== matlab function soc_dvbs2_fpga/DVBS2/DVBS2 TxRx/DVB-S2 HDL Receiver/Demod Deinterleave and FECDecode/Discard Unsupported Frames/convertMODCOD ==
  data: modcod input; modIdx output; codIdx output
function [modIdx,codIdx] = convertMODCOD(modcod)
%#codegen

     modIdx = fi(0,0,2,0,hdlfimath);
     codIdx = fi(0,0,4,0,hdlfimath);
     if modcod < 12
         modIdx(:) = 0;
     elseif modcod < 18
         modIdx(:) = 1;
     elseif modcod < 24
         modIdx(:) = 2;
     else
         modIdx(:) = 3;
     end

     switch modcod
         case 1
             codIdx(:) = 0; % 1/4
         case 2
             codIdx(:) =  1; % 1/3
         case 3
             codIdx(:) =  2; % 2/5
         case 4
             codIdx(:) =  3; % 1/2
         case {5,12}
             codIdx(:) =  4; % 3/5
         case {6,13,18}
             codIdx(:) =  5; % 2/3
         case {7,14,19,24}
             codIdx(:) =  6; % 3/4
         case {8,20,25}
             codIdx(:) =  7; % 4/5
         case {9,15,21,26}
             codIdx(:) =  8; % 5/6
         case {10,16,22,27}
             codIdx(:) =  9; % 8/9
         case {11,17,23,28}
             codIdx(:) = 10; % 9/10
         otherwise
             codIdx(:) = 0; % use this as default

     end
end

== matlab function soc_dvbs2_fpga/DVBS2/DVBS2 TxRx/DVB-S2 HDL Receiver/Stream Recovery/BB Decoder/Extract Data Field/Sample Discard Control ==
  data: dataIn input; dataOut output; startIn input; endIn input; validIn input; startOut output; endOut output; validOut output
function [dataOut,startOut,endOut,validOut] = SampleDiscardControl(dataIn,startIn,endIn,validIn)
%#codegen

persistent active dataOutReg startOutReg endOutReg validOutReg;
     if isempty(active)
         active       = false;
         dataOutReg   = cast(0,'like',dataIn);
         startOutReg  = false;
         endOutReg    = false;
         validOutReg  = false;
     end
     
     dataOut    = dataOutReg;
     startOut   = startOutReg;
     endOut     = endOutReg;
     validOut   = validOutReg;

     if startIn
         active = true;
     end

     if active && validIn
         dataOutReg = dataIn;
         validOutReg = true;
     else
         dataOutReg(:)  = 0;
         validOutReg = false;
     end

     if endIn
         active = false;
     end

     startOutReg = startIn;
     endOutReg = endIn;
     

end

== matlab function soc_dvbs2_fpga/DVBS2/DVBS2 TxRx/DVB-S2 HDL Receiver/Stream Recovery/BB Decoder/Extract Stream/Extract User Packet /Sample Discard Control ==
  data: dataIn input; dataOut output; startIn input; endIn input; validIn input; startOut output; endOut output; validOut output
function [dataOut,startOut,endOut,validOut] = SampleDiscardControl(dataIn,startIn,endIn,validIn)
%#codegen

persistent active dataOutReg startOutReg endOutReg validOutReg;
     if isempty(active)
         active         = false;
         dataOutReg     = dataIn;
         dataOutReg(:)  = 0;
         startOutReg    = false;
         endOutReg      = false;
         validOutReg    = false;
     end
     
     dataOut    = dataOutReg;
     startOut   = startOutReg;
     endOut     = endOutReg;
     validOut   = validOutReg;

     if startIn
         active = true;
     end

     if active && validIn
         dataOutReg = dataIn;
         validOutReg = true;
     else
         dataOutReg(:)  = 0;
         validOutReg = false;
     end

     if endIn
         active = false;
     end

     startOutReg = startIn;
     endOutReg = endIn;
     

end

== matlab function soc_dvbs2_fpga/DVBS2/DVBS2 TxRx/DVB-S2 HDL Receiver/Stream Recovery/BB Decoder/Extract Stream/Extract User Packet /Variable Count Limited HDL Counter ==
  data: rst input; countToValue input; enb input; Hit output
function Hit = VariableCountLimitedHDLCounter(rst,countToValue,enb)
%#codegen

    persistent countState;
    if isempty(countState)
        countState = cast(0,'like',countToValue);
    end
    
%     count = countState;
    if enb
        Hit0 = (countState == 0);
        HitcountToValue = (countState == countToValue - 1);
        Hit = [Hit0;HitcountToValue];
    else
        Hit = false(2,1);
    end

    if rst
        countState(:) = 0;
    elseif enb
        if countState == countToValue - 1
            countState(:) = 0;
        else
            countState(:) = countState + 1;
        end
    end
end

== matlab function soc_dvbs2_fpga/DVBS2/DVBS2 TxRx/DVB-S2 HDL Receiver/Demod Deinterleave and FECDecode/DVBS2 HDL Deinterleaver/Discard Out of  Frame samples ==
  data: dataIn input; dataOut output; valid input; validOut output; reset input; fec input
function [dataOut,validOut] = fcn(dataIn,valid,reset,fec)
%#codegen
  
  COUNTMAX_NORMAL = 64800;
  COUNTMAX_SHORT = 16200;

  persistent count dataReg validReg;
  if isempty(count)
      count = fi(COUNTMAX_NORMAL,0,nextpow2(COUNTMAX_NORMAL),0,hdlfimath);
      validReg = false;
      dataReg = cast(0,'like',dataIn);
  end
  
  dataOut = dataReg;
  validOut = validReg;

  if fec
      COUNTMAX = fi(COUNTMAX_SHORT,0,nextpow2(COUNTMAX_NORMAL),0,hdlfimath);
  else
      COUNTMAX = fi(COUNTMAX_NORMAL,0,nextpow2(COUNTMAX_NORMAL),0,hdlfimath);
  end


  if valid && (count < COUNTMAX)
      count(:) = count + 1;
      dataReg = dataIn;
      validReg = valid;
  else
      dataReg(:) = 0;
      validReg = false;
  end
  
  if reset
      count(:) = 0;
  end


end

== matlab function soc_dvbs2_fpga/DVBS2/DVBS2 TxRx/Channel/AWGN Generator/Unit Variance Gaussian Noise/SqrtImplementation/SqrtEval/RangeReduction/leadingZeroDetector ==
  data: x input; exp_f output
function exp_f=leadingZeroDetector(x)
%exp_e=31-length(dec2bin(x));
temp = 0;
flag=1.0e+09 *[

   0.000000002000000
   0.000000004000000
   0.000000008000000
   0.000000016000000
   0.000000032000000
   0.000000064000000
   0.000000128000000
   0.000000256000000
   0.000000512000000
   0.000001024000000
   0.000002048000000
   0.000004096000000
   0.000008192000000
   0.000016384000000
   0.000032768000000
   0.000065536000000
   0.000131072000000
   0.000262144000000
   0.000524288000000
   0.001048576000000
   0.002097152000000
   0.004194304000000
   0.008388608000000
   0.016777216000000
   0.033554432000000
   0.067108864000000
   0.134217728000000
   0.268435456000000
   0.536870912000000
   1.073741824000000
   2.147483648000000];

% else
%     while( )
%         temp = temp+1;
%         flag()=flag()*2;
%     end
% end
% 
% end
if(x == 0)
     temp = 31;
elseif (x*flag(1)>1)
        temp=1;
elseif (x*flag(2)>1)
        temp=2;
elseif (x*flag(3)>1)
        temp=3;
elseif (x*flag(4)>1)
        temp=4;
elseif (x*flag(5)>1)
        temp=5;
elseif (x*flag(6)>1)
        temp=6;
elseif (x*flag(7)>1)
        temp=7;
elseif (x*flag(8)>1)
        temp=8;
elseif (x*flag(9)>1)
        temp=9;
elseif (x*flag(10)>1)
        temp=10;
elseif (x*flag(11)>1)
        temp=11;
elseif (x*flag(12)>1)
        temp=12;
elseif (x*flag(13)>1)
        temp=13;
elseif (x*flag(14)>1)
        temp=14;
elseif (x*flag(15)>1)
        temp=15;
elseif (x*flag(16)>1)
        temp=16;
elseif (x*flag(17)>1)
        temp=17;
elseif (x*flag(18)>1)
        temp=18;
elseif (x*flag(19)>1)
        temp=19;
elseif (x*flag(20)>1)
        temp=20;
elseif (x*flag(21)>1)
        temp=21;
elseif (x*flag(22)>1)
        temp=22;
elseif (x*flag(23)>1)
        temp=23;
elseif (x*flag(24)>1)
        temp=24;
elseif (x*flag(25)>1)
        temp=25;
elseif (x*flag(26)>1)
        temp=26;
elseif (x*flag(27)>1)
        temp=27;
elseif (x*flag(28)>1)
        temp=28;
elseif (x*flag(29)>1)
        temp=29;
elseif (x*flag(30)>1)
        temp=30;              
end        
exp_f=uint8(temp);
